simulink model "PowerSupplySimulation"  (R2015b)
settings: Solver=VariableStepAuto  StartTime=0.0  StopTime=1  RelTol=1e-3
values from neighbouring files (symbols this model uses):
  c2_val = 200e-6    (= 0.0002)    [VoltageSourceController.m]    (also in main.m = 1e-06)
  fs1 = 2e3    (= 2000)    [CurrentSourceController.m]
  fs2 = 2e3    (= 2000)    [VoltageSourceController.m]
  l1_val = 500e-4    (= 0.05)    [CurrentSourceController.m]    (also in main.m = 4.8e-07)
  l2_val = 50e-4    (= 0.005)    [VoltageSourceController.m]    (also in main.m = 1e-08)
  r_val = 1    [CurrentSourceController.m]    (also in VoltageSourceController.m; main.m)
  rl1_val = 0.0002    [CurrentSourceController.m]    (also in main.m)
  Vd_val = 100    [CurrentSourceController.m]    (also in VoltageSourceController.m = 8; main.m = 110)
libraries: powerlib x23, simulink x2, simulink_extras x2
settings Model: Creator=Akshay  LastModifiedBy=Akshay

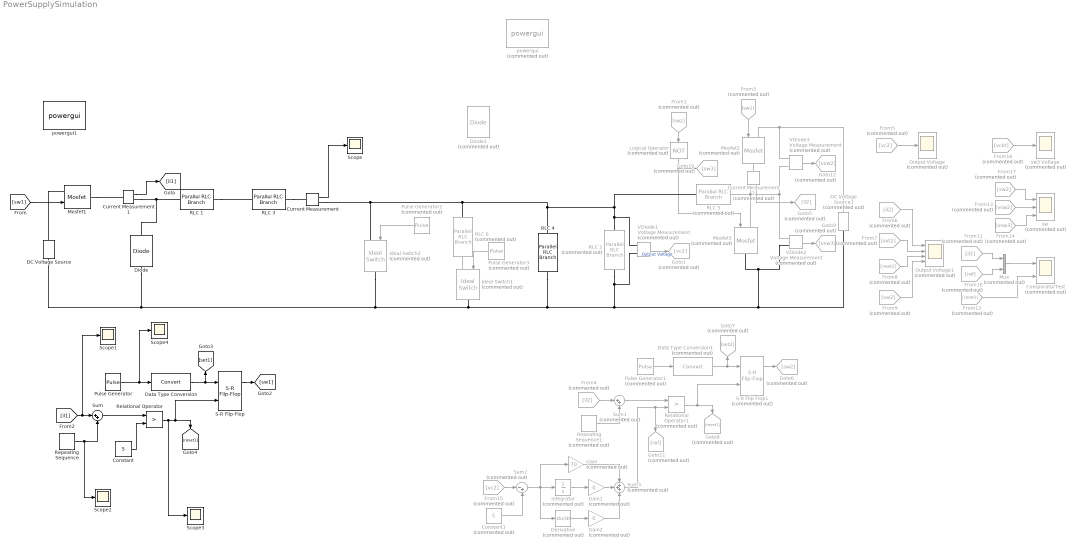
== system PowerSupplySimulation ==
  " RLC 1" : powerlib/Elements/Parallel RLC Branch  LConnTagsString=a  RConnTagsString=__new0  BranchType=R  Resistance=rl1_val  Inductance=5e-6  SetiL0=off  InitialCurrent=0  Capacitance=0.3e-6  Setx0=off  InitialVoltage=0  Measurements=None
  " RLC 2" : powerlib/Elements/Parallel RLC Branch  Commented=on  LConnTagsString=a  RConnTagsString=__new0  BranchType=C  Resistance=1  Inductance=1e-3  SetiL0=off  InitialCurrent=0  Capacitance=c2_val  Setx0=off  InitialVoltage=50  Measurements=None
  " RLC 3" : powerlib/Elements/Parallel RLC Branch  LConnTagsString=a  RConnTagsString=__new0  BranchType=L  Resistance=50  Inductance=l1_val  SetiL0=off  InitialCurrent=100  Capacitance=0.3e-6  Setx0=off  InitialVoltage=0  Measurements=None
  " RLC 4" : powerlib/Elements/Parallel RLC Branch  LConnTagsString=a  RConnTagsString=__new0  BranchType=R  Resistance=r_val  Inductance=1e-3  SetiL0=off  InitialCurrent=0  Capacitance=0.1e-6  Setx0=off  InitialVoltage=0  Measurements=None
  " RLC 5" : powerlib/Elements/Parallel RLC Branch  Commented=on  LConnTagsString=a  RConnTagsString=__new0  BranchType=L  Resistance=50  Inductance=l2_val  SetiL0=on  InitialCurrent=0  Capacitance=0.3e-6  Setx0=off  InitialVoltage=0  Measurements=None
  " RLC 6" : powerlib/Elements/Parallel RLC Branch  Commented=on  LConnTagsString=a  RConnTagsString=__new0  BranchType=R  Resistance=r_val  Inductance=1e-3  SetiL0=off  InitialCurrent=0  Capacitance=0.1e-6  Setx0=off  InitialVoltage=0  Measurements=None
  ComparatorTest : Scope  Commented=on  NumInputPorts=2
  Constant : Constant  Value=5
  Constant1 : Constant  Commented=on  Value=5
  Current Measurement : powerlib/Measurements/Current Measurement  PhasorSimulation=off  OutputType=Complex  PSBequivalent=0
  Current Measurement1 : powerlib/Measurements/Current Measurement  PhasorSimulation=off  OutputType=Complex  PSBequivalent=0
  Current Measurement2 : powerlib/Measurements/Current Measurement  Commented=on  PhasorSimulation=off  OutputType=Complex  PSBequivalent=0
  DC Voltage Source : powerlib/Electrical Sources/DC Voltage Source  Amplitude=Vd_val  Measurements=Voltage
  DC Voltage Source1 : powerlib/Electrical Sources/DC Voltage Source  Commented=on  Amplitude=Vd_val  Measurements=Voltage
  Data Type Conversion : DataTypeConversion
  Data Type Conversion1 : DataTypeConversion  Commented=on
  Derivative : Derivative  Commented=on
  Diode : powerlib/Power Electronics/Diode  Ron=0.001  Lon=0  Vf=0.8  IC=0  UseSnubber=off  Rs=500  Cs=250e-9  Measurements=off
  Diode1 : powerlib/Power Electronics/Diode  Commented=on  Ron=0.001  Lon=0  Vf=0.8  IC=0  UseSnubber=off  Rs=500  Cs=250e-9  Measurements=on
  From{1,3,9,17} (4 alike) : From  Commented=on  GotoTag=sw2
  From10 : From  Commented=on  GotoTag=ref
  From11 : From  Commented=on  GotoTag=il2
  From12 : From  Commented=on  GotoTag=reset2
  From13 : From  Commented=on  GotoTag=vsw2
  From14 : From  Commented=on  GotoTag=vsw3
  From15 : From  Commented=on  GotoTag=vc2
  From16 : From  Commented=on  GotoTag=vckt
  From4 : From  Commented=on  GotoTag=il2
  From5 : From  Commented=on  GotoTag=vc2
  From6 : From  Commented=on  GotoTag=il2
  From7 : From  Commented=on  GotoTag=set2
  From8 : From  Commented=on  GotoTag=reset2
  Gain : Gain  Commented=on  Gain=70
  Gain1 : Gain  Commented=on  Gain=0
  Gain2 : Gain  Commented=on  Gain=0
  Goto1 : Goto  Commented=on  GotoTag=vc2
  Goto10 : Goto  Commented=on  GotoTag=sw3
  Goto11 : Goto  Commented=on  GotoTag=ref
  Goto12 : Goto  Commented=on  GotoTag=vsw2
  Goto5 : Goto  Commented=on  GotoTag=il2
  Goto6 : Goto  Commented=on  GotoTag=sw2
  Goto7 : Goto  Commented=on  GotoTag=set2
  Goto8 : Goto  Commented=on  GotoTag=reset2
  Goto9 : Goto  Commented=on  GotoTag=vsw3
  Ideal Switch1 : powerlib/Power Electronics/Ideal Switch  Commented=on  Ron=1e-7  Lon=0  IC=0  Rs=inf  Cs=inf  Measurements=off
  Ideal Switch2 : powerlib/Power Electronics/Ideal Switch  Commented=on  Ron=1e-7  Lon=0  IC=0  Rs=inf  Cs=inf  Measurements=off
  Integrator : Integrator  Commented=on  ZeroCross=off
  Logical Operator : Logic  Commented=on  Operator=NOT  AllPortsSameDT=off  OutDataTypeStr=boolean
  Mosfet1 : powerlib/Power Electronics/Mosfet  Ron=0.00001  Lon=0  Rd=0.0000000000001  Vfd=0  IC=0  Rs=1e5  Cs=inf  Measurements=off
  Mosfet2 : powerlib/Power Electronics/Mosfet  Commented=on  Ron=0.00001  Lon=0  Rd=0.0000000000001  Vfd=0  IC=0  Rs=1e5  Cs=inf  Measurements=off
  Mosfet3 : powerlib/Power Electronics/Mosfet  Commented=on  Ron=0.00001  Lon=0  Rd=0.0000000000001  Vfd=0  IC=0  Rs=1e5  Cs=inf  Measurements=off
  Mux : Mux  Commented=on  Inputs=2
  Output Voltage : Scope  Commented=on
  Output Voltage1 : Scope  Commented=on  NumInputPorts=4
  Pulse Generator : DiscretePulseGenerator  PulseType=Time based  Period=1/fs1  PulseWidth=5
  Pulse Generator1 : DiscretePulseGenerator  Commented=on  PulseType=Time based  Period=1/fs2  PulseWidth=5
  Pulse Generator2 : DiscretePulseGenerator  Commented=on  PulseType=Time based  Period=1/100  PulseWidth=90  PhaseDelay=0.1/100
  Pulse Generator3 : DiscretePulseGenerator  Commented=on  PulseType=Time based  Period=1/100  PulseWidth=90  PhaseDelay=0.05/100
  Relational Operator : RelationalOperator  Operator=>  OutDataTypeStr=boolean  ZeroCross=off
  Relational Operator1 : RelationalOperator  Commented=on  Operator=>  OutDataTypeStr=boolean  ZeroCross=off
  Repeating Sequence : simulink/Sources/Repeating Sequence  rep_seq_t=[0 1/fs1]  rep_seq_y=[0 0]
  Repeating Sequence1 : simulink/Sources/Repeating Sequence  Commented=on  rep_seq_t=[0 1/fs2]  rep_seq_y=[0 0]
  S-R Flip-Flop : simulink_extras/Flip Flops/S-R Flip-Flop  initial_condition=0
  S-R Flip-Flop1 : simulink_extras/Flip Flops/S-R Flip-Flop  Commented=on  initial_condition=0
  Scope{,1..4} (5 alike) : Scope
  Sum : Sum  Inputs=|++
  Sum1 : Sum  Commented=on  Inputs=|++
  Sum2 : Sum  Commented=on  Inputs=|-+
  Sum3 : Sum  Commented=on  Inputs=+++
  VDiode1 : powerlib/Measurements/Voltage Measurement  Commented=on  PhasorSimulation=off  OutputType=Complex  PSBequivalent=0
  VDiode2 : powerlib/Measurements/Voltage Measurement  Commented=on  PhasorSimulation=off  OutputType=Complex  PSBequivalent=0
  VDiode3 : powerlib/Measurements/Voltage Measurement  Commented=on  PhasorSimulation=off  OutputType=Complex  PSBequivalent=0
  powergui : powerlib/powergui  Priority=1  Commented=on  SimulationMode=Continuous  SolverType=Backward Euler  SampleTime=5e-07  frequency=60  SPID=on  DisableSnubberDevices=off  DisableRonSwitches=off  DisableVfSwitches=off  SwTol=0  DisplayEquations=off  Interpol=off  ExternalGateDelay=off  methode=off  Ts=0  FunctionMessages=off  echomessages=off  HookPort=off  EnableUseOfTLC=off  x0status=zero  frequencyindice=0  Pbase=100e6  ErrMax=1e-4  Iterations=50  UnitsV=kV  UnitsW=MW  buscounter=0  RestoreLinks=warning  ResistiveCurrentMeasurement=off  Frange=[0:2:500]  Ylog=off  Xlog=on  ShowGrid=off  save=off  variable=ZData  structure=ScopeData  ZoomFFT=off  StartTime=0.0  cycles=5  DisplayStyle=2  fundamental=50  FreqAxis=off  MaxFrequency=50000  frequencyindicesteady=1  RmsSteady=1  display=off
  powergui1 : powerlib/powergui  Priority=1  SimulationMode=Continuous  SolverType=Backward Euler  SampleTime=5e-07  frequency=60  SPID=on  DisableSnubberDevices=off  DisableRonSwitches=off  DisableVfSwitches=off  SwTol=0  DisplayEquations=off  Interpol=off  ExternalGateDelay=off  methode=off  Ts=0  FunctionMessages=off  echomessages=off  HookPort=off  EnableUseOfTLC=off  x0status=zero  frequencyindice=0  Pbase=100e6  ErrMax=1e-4  Iterations=50  UnitsV=kV  UnitsW=MW  buscounter=0  RestoreLinks=warning  ResistiveCurrentMeasurement=off  Frange=[0:2:500]  Ylog=off  Xlog=on  ShowGrid=off  save=off  variable=ZData  structure=ScopeData  ZoomFFT=off  StartTime=0.0  cycles=5  DisplayStyle=2  fundamental=50  FreqAxis=off  MaxFrequency=50000  frequencyindicesteady=1  RmsSteady=1  display=off
  sw : Scope  Commented=on  NumInputPorts=3
  sw3 Voltage : Scope  Commented=on
  wires:
  Current Measurement/1 -> Scope/1
  Pulse Generator/1 -> Scope4/1, Data Type Conversion/1
  Data Type Conversion/1 -> S-R Flip-Flop/1, [set1]
  Relational Operator/1 -> Scope3/1, S-R Flip-Flop/2, [reset1]
  S-R Flip-Flop/1 -> [sw1]
  [il1] -> Scope1/1, Sum/1
  Repeating Sequence/1 -> Scope2/1, Sum/2
  Sum/1 -> Relational Operator/1
  Current Measurement1/1 -> [il1]
  Constant/1 -> Relational Operator/2
  [sw1] -> Mosfet1/1
  VDiode1/1 -> Goto1/1  "Output Voltage"
  Current Measurement2/1 -> Goto5/1
  Pulse Generator1/1 -> Data Type Conversion1/1
  Data Type Conversion1/1 -> S-R Flip-Flop1/1, Goto7/1
  From1/1 -> Logical Operator/1
  Relational Operator1/1 -> S-R Flip-Flop1/2, Goto8/1
  From5/1 -> Output Voltage/1
  From6/1 -> Output Voltage1/1
  From7/1 -> Output Voltage1/2
  From8/1 -> Output Voltage1/3
  From9/1 -> Output Voltage1/4
  VDiode2/1 -> Goto9/1
  From16/1 -> sw3 Voltage/1
  From17/1 -> sw/1
  S-R Flip-Flop1/1 -> Goto6/1
  Logical Operator/1 -> Goto10/1, Mosfet3/1
  From11/1 -> Mux/1
  From10/1 -> Mux/2
  Mux/1 -> ComparatorTest/1
  From12/1 -> ComparatorTest/2
  VDiode3/1 -> Goto12/1
  From14/1 -> sw/3
  From13/1 -> sw/2
  From4/1 -> Sum1/1
  Repeating Sequence1/1 -> Sum1/2
  Sum1/1 -> Relational Operator1/1
  From15/1 -> Sum2/1
  Constant1/1 -> Sum2/2
  Sum2/1 -> Derivative/1, Gain/1, Integrator/1
  Integrator/1 -> Gain1/1
  Gain1/1 -> Sum3/2
  Gain/1 -> Sum3/1
  Sum3/1 -> Relational Operator1/2, Goto11/1
  Derivative/1 -> Gain2/1
  Gain2/1 -> Sum3/3
  From3/1 -> Mosfet2/1
  Pulse Generator2/1 -> Ideal Switch2/1
  Pulse Generator3/1 -> Ideal Switch1/1
  connections:
  Current Measurement1/RConn1 -- Diode/RConn1 -- " RLC 1"/LConn1
  " RLC 1"/RConn1 -- " RLC 3"/LConn1
  Mosfet1/RConn1 -- Current Measurement1/LConn1
  DC Voltage Source/RConn1 -- Mosfet1/LConn1
  " RLC 3"/RConn1 -- Current Measurement/LConn1
  Mosfet3/LConn1 -- VDiode3/LConn2 -- VDiode2/LConn1 -- " RLC 5"/RConn1 -- Current Measurement2/RConn1
  DC Voltage Source/LConn1 -- Diode/LConn1 -- Ideal Switch2/RConn1 -- Ideal Switch1/RConn1 -- Mosfet3/RConn1 -- VDiode2/LConn2 -- DC Voltage Source1/LConn1 -- " RLC 2"/RConn1 -- VDiode1/LConn2 -- " RLC 4"/RConn1
  VDiode3/LConn1 -- Mosfet2/LConn1 -- DC Voltage Source1/RConn1
  Mosfet2/RConn1 -- Current Measurement2/LConn1
  Current Measurement/RConn1 -- Ideal Switch2/LConn1 -- " RLC 4"/LConn1 -- " RLC 5"/LConn1 -- " RLC 2"/LConn1 -- VDiode1/LConn1 -- " RLC 6"/LConn1
  Ideal Switch1/LConn1 -- " RLC 6"/RConn1
